simulink model "modelo_ARMAX"  (R2015a)
settings: Solver=ode45  StartTime=0.0  StopTime=200  RelTol=1e-3
values from neighbouring files (symbols this model uses):
  lambda = 1    [generar_prbs.m]    (also in parametros_ident.m = 0.995)
undefined symbols (not defined in the file or in its folder): sigbuilder_block
settings Model: Creator=u_labelectro  LastModifiedBy=Luis
settings DebuggingCC: UnderspecifiedInitializationDetection=Classic  MergeDetectMultiDrivingBlocksExec=none  SolverPrmCheckMsg=warning  StateNameClashWarn=warning

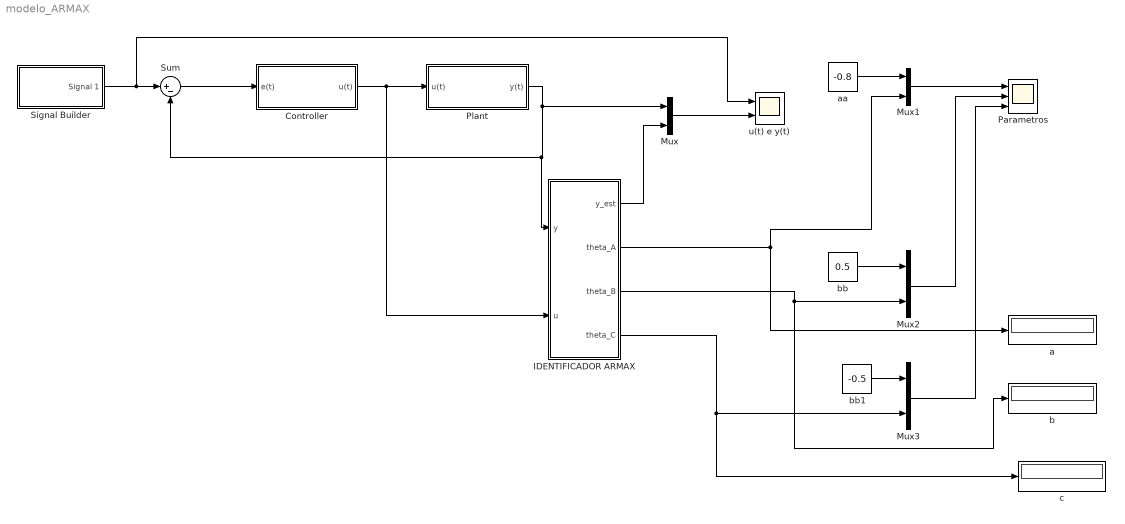
== system modelo_ARMAX ==
  Controller : Subsystem
  IDENTIFICADOR ARMAX : Subsystem
  Mux{,1..3} (4 alike) : Mux  Inputs=2
  Parametros : Scope  NumInputPorts=3
      settings: YMin=-5~-5~-5  YMax=5~5~5
  Plant : Subsystem
  Signal Builder : Subsystem  Tag=STV Subsys  LoadFcn=sigbuilder_block('load');  StartFcn=sigbuilder_block('start');  StopFcn=sigbuilder_block('stop');  ClipboardFcn=sigbuilder_block('clipboard');  mask(Sigbuilder block){}
      mask help: Simulink:masks:SigbuilderBlock_MD
      mask init:
      | if ~strcmp(get_param(bdroot(gcbh),'SimulationStatus'),'stopped') tuvar = sigbuilder_block('maskInit'); end
      settings: CopyFcn=sigbuilder_block('copy');  DeleteFcn=sigbuilder_block('delete');  ModelCloseFcn=sigbuilder_block('modelClose');  PreSaveFcn=sigbuilder_block('preSave');  PauseFcn=sigbuilder_block('pause');  ContinueFcn=sigbuilder_block('continue');  NameChangeFcn=sigbuilder_block('namechange');  OpenFcn=sigbuilder_block('open',[0 30 1080 588 ]);  CloseFcn=sigbuilder_block('close');
      mask Display: plot(0, 0, 100, 100,[2, 2, 32, 32, 2], [68, 8, 8, 68, 68],[32, 2], [38, 38], [32, 19, 2],[53, 60, 44], [32, 17, 17, 2],[16, 16, 31, 31]);txt = getActiveGroup(gcbh);text(2, 100, txt,'verticalAlignment', 'top');
  Sum : Sum  Inputs=|+-
  a : Display
  aa : Constant  Value=-0.8
  b : Display
  bb : Constant  Value=0.5
  bb1 : Constant  Value=-0.5
  c : Display
  u(t) e y(t) : Scope  NumInputPorts=2
      settings: YMin=-5~-5  YMax=5~5
  wires:
  Signal Builder/1(Signal 1) -> u(t) e y(t)/1, Sum/1
  Sum/1 -> Controller/1(e(t))
  Controller/1(u(t)) -> IDENTIFICADOR ARMAX/2(u), Plant/1(u(t))
  Plant/1(y(t)) -> Mux/1, IDENTIFICADOR ARMAX/1(y), Sum/2
  IDENTIFICADOR ARMAX/1(y_est) -> Mux/2
  Mux/1 -> u(t) e y(t)/2
  aa/1 -> Mux1/1
  IDENTIFICADOR ARMAX/2(theta_A) -> Mux1/2, a/1
  bb/1 -> Mux2/1
  IDENTIFICADOR ARMAX/3(theta_B) -> b/1, Mux2/2
  Mux1/1 -> Parametros/1
  Mux2/1 -> Parametros/2
  IDENTIFICADOR ARMAX/4(theta_C) -> Mux3/2, c/1
  bb1/1 -> Mux3/1
  Mux3/1 -> Parametros/3

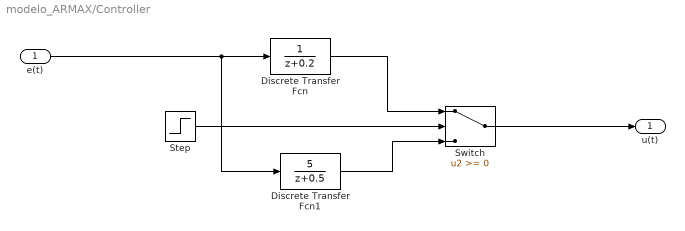
== system modelo_ARMAX/Controller ==
  e(t) : Inport
  Discrete Transfer Fcn : DiscreteTransferFcn  Denominator=[1 0.2]  SampleTime=0.01
  Discrete Transfer Fcn1 : DiscreteTransferFcn  Numerator=[5]  SampleTime=0.01
  Step : Step  Time=50  SampleTime=0
  Switch : Switch
  u(t) : Outport
  wires:
  Step/1 -> Switch/2
  Discrete Transfer Fcn1/1 -> Switch/3
  Discrete Transfer Fcn/1 -> Switch/1
  e(t)/1 -> Discrete Transfer Fcn1/1, Discrete Transfer Fcn/1
  Switch/1 -> u(t)/1

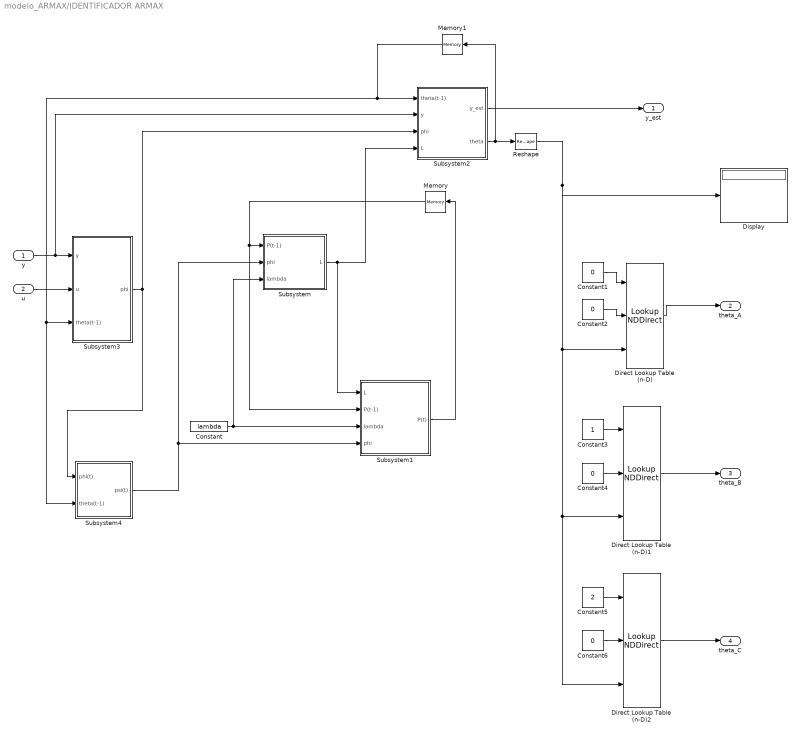
== system modelo_ARMAX/IDENTIFICADOR ARMAX ==
  y : Inport
  u : Inport  Port=2
  Constant : Constant  Value=lambda
  Constant{1..2,4,6} (4 alike) : Constant  Value=0
  Constant3 : Constant
  Constant5 : Constant  Value=2
  Direct Lookup Table (n-D) : LookupNDDirect  TableIsInput=on  Table=[4 5 ;16 19 ]  DiagnosticForOutOfRangeInput=Error  SampleTime=0.01
  Direct Lookup Table (n-D)1 : LookupNDDirect  TableIsInput=on  Table=[4 5 ;16 19 ]  DiagnosticForOutOfRangeInput=Error  SampleTime=0.01
  Direct Lookup Table (n-D)2 : LookupNDDirect  TableIsInput=on  Table=[4 5 ;16 19 ]  DiagnosticForOutOfRangeInput=Error  SampleTime=0.01
  Display : Display
  Memory : Memory  X0=1e6*eye(3)
  Memory1 : Memory
  Reshape : Reshape  OutputDimensionality=Column vector (2-D)
  Subsystem : Subsystem
  Subsystem1 : Subsystem
  Subsystem2 : Subsystem
  Subsystem3 : Subsystem
  Subsystem4 : Subsystem
  y_est : Outport
  theta_A : Outport  Port=2
  theta_B : Outport  Port=3
  theta_C : Outport  Port=4
  wires:
  y/1 -> Subsystem2/2(y), Subsystem3/1(y)
  Subsystem3/1(phi) -> Subsystem2/3(phi), Subsystem4/1(phi(t))
  Subsystem/1(L) -> Subsystem1/1(L), Subsystem2/4(L)
  u/1 -> Subsystem3/2(u)
  Constant/1 -> Subsystem1/3(lambda), Subsystem/3(lambda)
  Subsystem1/1(P(t)) -> Memory/1
  Memory/1 -> Subsystem1/2(P(t-1)), Subsystem/1(P(t-1))
  Subsystem2/1(y_est) -> y_est/1
  Subsystem2/2(theta) -> Reshape/1, Memory1/1
  Memory1/1 -> Subsystem4/2(theta(t-1)), Subsystem3/3(theta(t-1)), Subsystem2/1(theta(t-1))
  Constant4/1 -> Direct Lookup Table (n-D)1/2
  Constant3/1 -> Direct Lookup Table (n-D)1/1
  Constant1/1 -> Direct Lookup Table (n-D)/1
  Direct Lookup Table (n-D)/1 -> theta_A/1
  Direct Lookup Table (n-D)1/1 -> theta_B/1
  Constant2/1 -> Direct Lookup Table (n-D)/2
  Constant6/1 -> Direct Lookup Table (n-D)2/2
  Constant5/1 -> Direct Lookup Table (n-D)2/1
  Direct Lookup Table (n-D)2/1 -> theta_C/1
  Reshape/1 -> Direct Lookup Table (n-D)/3, Direct Lookup Table (n-D)2/3, Direct Lookup Table (n-D)1/3, Display/1
  Subsystem4/1(psi(t)) -> Subsystem1/4(phi), Subsystem/2(phi)

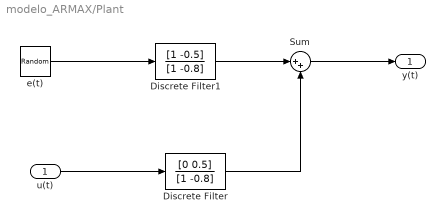
== system modelo_ARMAX/Plant ==
  u(t) : Inport
  Discrete Filter : DiscreteFilter  Numerator=[0 0.5]  Denominator=[1 -0.8]  SampleTime=0.01
  Discrete Filter1 : DiscreteFilter  Numerator=[1 -0.5]  Denominator=[1 -0.8]
  Sum : Sum  Inputs=|++
  e(t) : RandomNumber  Variance=0.00001  SampleTime=0.1
  y(t) : Outport
  wires:
  Discrete Filter/1 -> Sum/2
  Discrete Filter1/1 -> Sum/1
  Sum/1 -> y(t)/1
  u(t)/1 -> Discrete Filter/1
  e(t)/1 -> Discrete Filter1/1

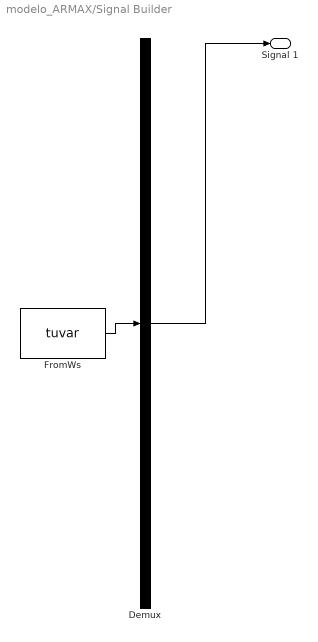
== system modelo_ARMAX/Signal Builder ==
  Demux : Demux  Tag=STV Demux  Outputs=1
  FromWs : FromWorkspace  Tag=STV FromWs  VariableName=tuvar  SampleTime=0
      SigBuilderData=|
      | common.afterFinalStr = 'Extrapolate'
      | common.sampleTime = 0
      | dataSet.timeRange = [0 10]
      | dataSet.name = 'Group 1'
      | sbobj.Groups.Name = 'Group 1'
      | sbobj.Groups.Signals.Name = 'Signal 1'
      | sbobj.Groups.Signals.XData = [0 3.18 3.18 6 6 10]
      | sbobj.Groups.Signals.YData = [0 0 0.455 0.455 0.845 0.845]
  Signal 1 : Outport  Tag=STV Outport
  wires:
  Demux/1 -> Signal 1/1
  FromWs/1 -> Demux/1

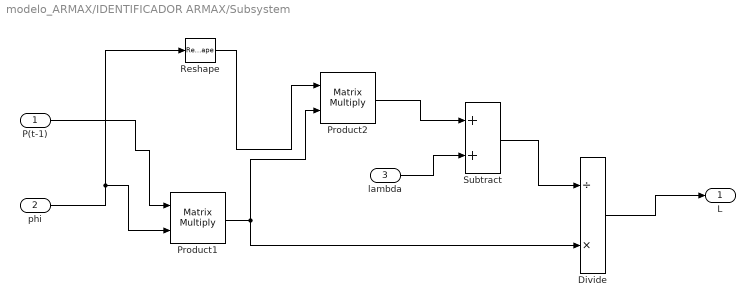
== system modelo_ARMAX/IDENTIFICADOR ARMAX/Subsystem ==
  P(t-1) : Inport
  phi : Inport  Port=2
  lambda : Inport  Port=3
  Divide : Product  Inputs=/*
  Product1 : Product  Multiplication=Matrix(*)  SampleTime=0.01
  Product2 : Product  Multiplication=Matrix(*)  SampleTime=0.01
  Reshape : Reshape  OutputDimensionality=Row vector (2-D)
  Subtract : Sum
  L : Outport
  wires:
  Divide/1 -> L/1
  Subtract/1 -> Divide/1
  phi/1 -> Product1/2, Reshape/1
  Reshape/1 -> Product2/1
  lambda/1 -> Subtract/2
  Product1/1 -> Divide/2, Product2/2
  P(t-1)/1 -> Product1/1
  Product2/1 -> Subtract/1

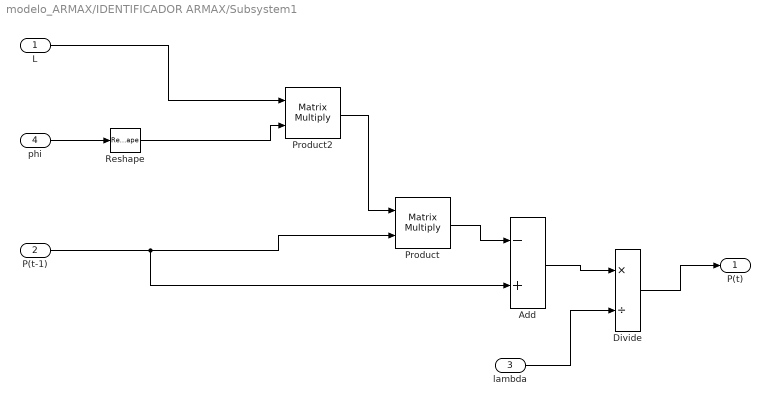
== system modelo_ARMAX/IDENTIFICADOR ARMAX/Subsystem1 ==
  L : Inport
  P(t-1) : Inport  Port=2
  lambda : Inport  Port=3
  phi : Inport  Port=4
  Add : Sum  Inputs=-+
  Divide : Product  Inputs=*/
  Product : Product  Multiplication=Matrix(*)  SampleTime=0.01
  Product2 : Product  Multiplication=Matrix(*)  SampleTime=0.01
  Reshape : Reshape  OutputDimensionality=Row vector (2-D)
  P(t) : Outport
  wires:
  L/1 -> Product2/1
  phi/1 -> Reshape/1
  Reshape/1 -> Product2/2
  Product2/1 -> Product/1
  P(t-1)/1 -> Product/2, Add/2
  Product/1 -> Add/1
  Add/1 -> Divide/1
  Divide/1 -> P(t)/1
  lambda/1 -> Divide/2

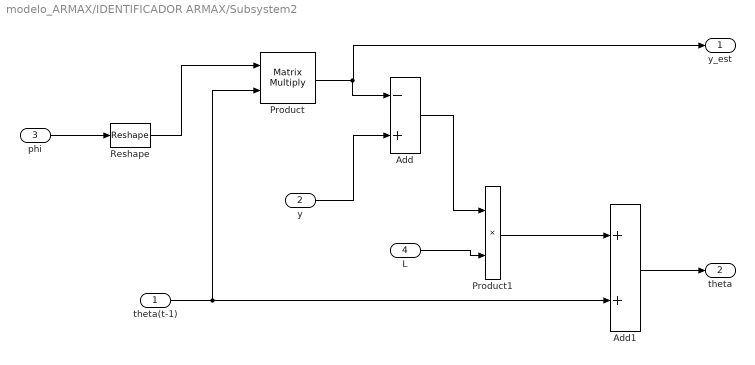
== system modelo_ARMAX/IDENTIFICADOR ARMAX/Subsystem2 ==
  theta(t-1) : Inport
  y : Inport  Port=2
  phi : Inport  Port=3
  L : Inport  Port=4
  Add : Sum  Inputs=-+
  Add1 : Sum
  Product : Product  Multiplication=Matrix(*)  SampleTime=0.01
  Product1 : Product
  Reshape : Reshape  OutputDimensionality=Row vector (2-D)
  y_est : Outport
  theta : Outport  Port=2
  wires:
  Product/1 -> Add/1, y_est/1
  y/1 -> Add/2
  L/1 -> Product1/2
  Add/1 -> Product1/1
  Product1/1 -> Add1/1
  Add1/1 -> theta/1
  theta(t-1)/1 -> Product/2, Add1/2
  Reshape/1 -> Product/1
  phi/1 -> Reshape/1

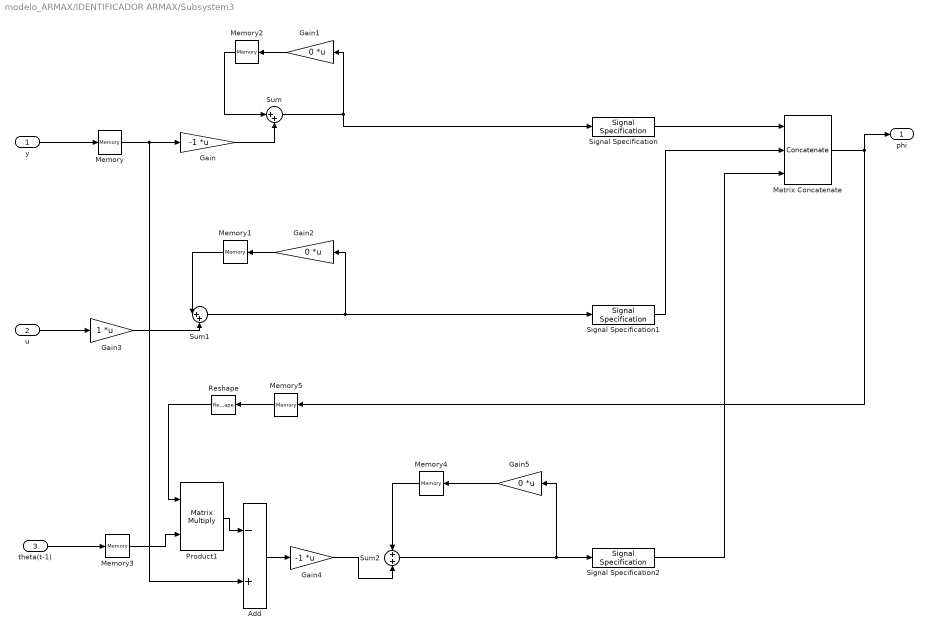
== system modelo_ARMAX/IDENTIFICADOR ARMAX/Subsystem3 ==
  y : Inport
  u : Inport  Port=2
  theta(t-1) : Inport  Port=3
  Add : Sum  Inputs=-+
  Gain : Gain  Gain=-1  Multiplication=Matrix(K*u)
  Gain1 : Gain  Gain=0  Multiplication=Matrix(K*u)
  Gain2 : Gain  Gain=0  Multiplication=Matrix(K*u)
  Gain3 : Gain  Multiplication=Matrix(K*u)
  Gain4 : Gain  Gain=-1  Multiplication=Matrix(K*u)
  Gain5 : Gain  Gain=0  Multiplication=Matrix(K*u)
  Matrix Concatenate : Concatenate  NumInputs=3  Mode=Multidimensional array
  Memory{,1..5} (6 alike) : Memory
  Product1 : Product  Multiplication=Matrix(*)  SampleTime=0.01
  Reshape : Reshape  OutputDimensionality=Row vector (2-D)
  Signal Specification : SignalSpecification  Dimensions=[1 1]
  Signal Specification1 : SignalSpecification  Dimensions=[1 1]
  Signal Specification2 : SignalSpecification  Dimensions=[1 1]
  Sum : Sum  Inputs=|++
  Sum1 : Sum  Inputs=|++
  Sum2 : Sum
  phi : Outport
  wires:
  Sum/1 -> Gain1/1, Signal Specification/1
  Gain1/1 -> Memory2/1
  Memory2/1 -> Sum/1
  Gain/1 -> Sum/2
  Memory/1 -> Add/2, Gain/1
  y/1 -> Memory/1
  Gain2/1 -> Memory1/1
  u/1 -> Gain3/1
  Gain3/1 -> Sum1/2
  Memory1/1 -> Sum1/1
  Sum1/1 -> Gain2/1, Signal Specification1/1
  Signal Specification/1 -> Matrix Concatenate/1
  Signal Specification1/1 -> Matrix Concatenate/2
  Matrix Concatenate/1 -> phi/1, Memory5/1
  theta(t-1)/1 -> Memory3/1
  Reshape/1 -> Product1/1
  Memory5/1 -> Reshape/1
  Memory3/1 -> Product1/2
  Add/1 -> Gain4/1
  Gain4/1 -> Sum2/2
  Memory4/1 -> Sum2/1
  Gain5/1 -> Memory4/1
  Sum2/1 -> Gain5/1, Signal Specification2/1
  Signal Specification2/1 -> Matrix Concatenate/3
  Product1/1 -> Add/1

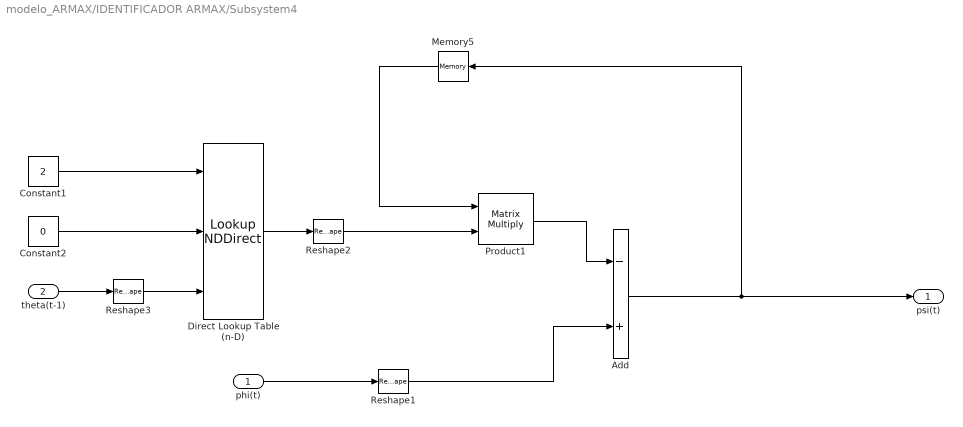
== system modelo_ARMAX/IDENTIFICADOR ARMAX/Subsystem4 ==
  phi(t) : Inport
  theta(t-1) : Inport  Port=2
  Add : Sum  Inputs=-+
  Constant1 : Constant  Value=2
  Constant2 : Constant  Value=0
  Direct Lookup Table (n-D) : LookupNDDirect  TableIsInput=on  Table=[4 5 ;16 19 ]  DiagnosticForOutOfRangeInput=Error  SampleTime=0.01
  Memory5 : Memory
  Product1 : Product  Multiplication=Matrix(*)  SampleTime=0.01
  Reshape1 : Reshape  OutputDimensionality=Column vector (2-D)
  Reshape2 : Reshape  OutputDimensionality=Column vector (2-D)
  Reshape3 : Reshape  OutputDimensionality=Column vector (2-D)
  psi(t) : Outport
  wires:
  Memory5/1 -> Product1/1
  Add/1 -> Memory5/1, psi(t)/1
  phi(t)/1 -> Reshape1/1
  Reshape1/1 -> Add/2
  Reshape2/1 -> Product1/2
  theta(t-1)/1 -> Reshape3/1
  Constant1/1 -> Direct Lookup Table (n-D)/1
  Constant2/1 -> Direct Lookup Table (n-D)/2
  Direct Lookup Table (n-D)/1 -> Reshape2/1
  Reshape3/1 -> Direct Lookup Table (n-D)/3
  Product1/1 -> Add/1
